simulink model "pid_controller"  (R2022a)
settings: Solver=VariableStepAuto  StartTime=0.0  StopTime=10.0  RelTol=1e-3
undefined symbols (not defined in the file): Kd, Ki, Kp
settings Model: Creator=stakk  LastModifiedBy=stakk

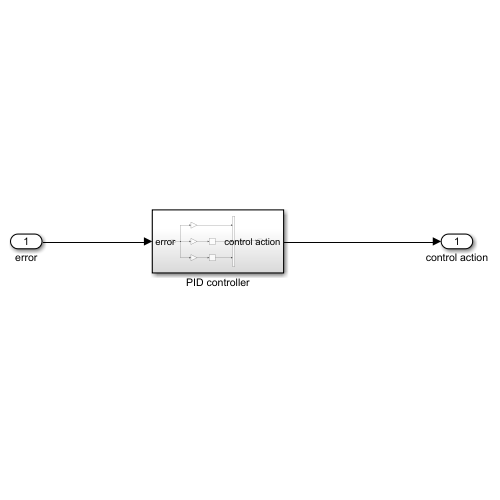
[thumbnail: Simulink's stored preview of the top-level diagram]
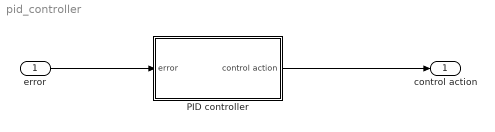
== system pid_controller ==
  error : Inport
  PID controller : Subsystem
  control action : Outport
  wires:
  error/1 -> PID controller/1(error)
  PID controller/1(control action) -> control action/1

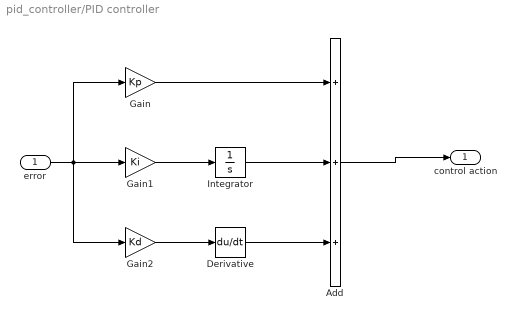
== system pid_controller/PID controller ==
  error : Inport
  Add : Sum  Inputs=+++
  Derivative : Derivative
  Gain : Gain  Gain=Kp
  Gain1 : Gain  Gain=Ki
  Gain2 : Gain  Gain=Kd
  Integrator : Integrator
  control action : Outport
  wires:
  Integrator/1 -> Add/2
  Add/1 -> control action/1
  Derivative/1 -> Add/3
  error/1 -> Gain/1, Gain2/1, Gain1/1
  Gain/1 -> Add/1
  Gain2/1 -> Derivative/1
  Gain1/1 -> Integrator/1
